simulink model "motorFFT"  (R2024b)
settings: Solver=FixedStepAuto  StartTime=0.0  StopTime=64  FixedStep=15e-3  RelTol=1e-3
libraries: SignalEditorBlockLib x9, spspowerguiLib x1
settings Model: SimulationMode=rapid-accelerator  Creator=Nitesh  LastModifiedBy=Nitesh
settings DataIOCC: ReturnWorkspaceOutputs=off
settings GRTTargetCC: RTWCAPISignals=on  RTWCAPIParams=on

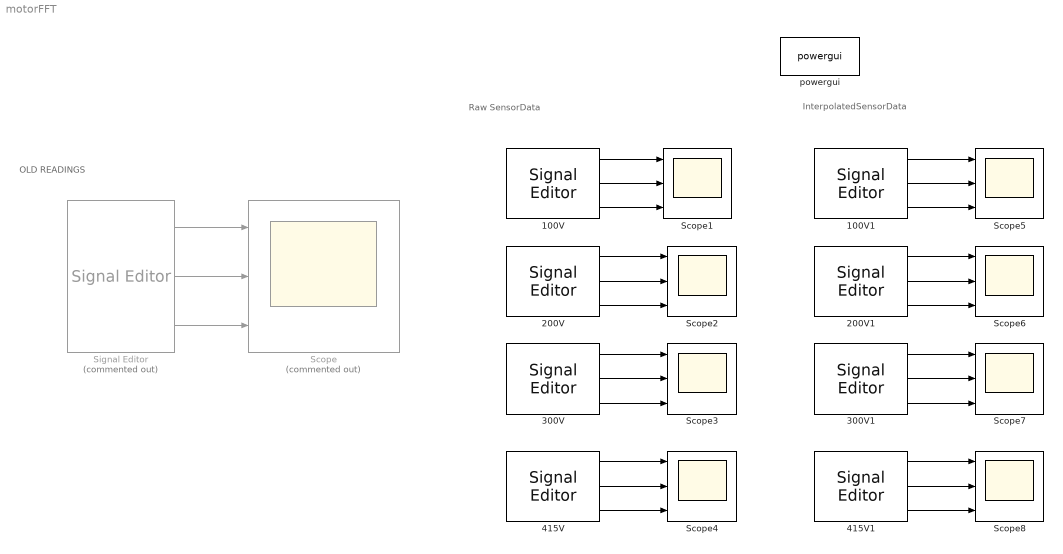
== system motorFFT ==
  note: InterpolatedSensorData
  note: Raw SensorData
  note: OLD READINGS
  100V : SignalEditorBlockLib/Signal Editor  FileName=_100V_scenario.mat  ActiveScenario=scenario  ActiveSignal=Xa  IsBus=off  OutputBusObjectStr=Bus: BusObject  SampleTime=0  Interpolate=off  ZeroCross=off  OutputAfterFinalValue=Setting to zero  Unit=inherit  PreserveSignalName=on  ApplySigPropsToAllScenarios=on  ApplySigPropsToAllSignals=on
  100V1 : SignalEditorBlockLib/Signal Editor  FileName=_100V_scenario.mat  ActiveScenario=scenario  ActiveSignal=Xa  IsBus=off  OutputBusObjectStr=Bus: BusObject  SampleTime=0  ZeroCross=off  OutputAfterFinalValue=Setting to zero  Unit=inherit  PreserveSignalName=on  ApplySigPropsToAllScenarios=on  ApplySigPropsToAllSignals=on
  200V : SignalEditorBlockLib/Signal Editor  FileName=_200V_scenario.mat  ActiveScenario=scenario  ActiveSignal=Xa  IsBus=off  OutputBusObjectStr=Bus: BusObject  SampleTime=0  Interpolate=off  ZeroCross=off  OutputAfterFinalValue=Setting to zero  Unit=inherit  PreserveSignalName=on  ApplySigPropsToAllScenarios=on  ApplySigPropsToAllSignals=on
  200V1 : SignalEditorBlockLib/Signal Editor  FileName=_200V_scenario.mat  ActiveScenario=scenario  ActiveSignal=Xa  IsBus=off  OutputBusObjectStr=Bus: BusObject  SampleTime=0  ZeroCross=off  OutputAfterFinalValue=Setting to zero  Unit=inherit  PreserveSignalName=on  ApplySigPropsToAllScenarios=on  ApplySigPropsToAllSignals=on
  300V : SignalEditorBlockLib/Signal Editor  FileName=_300_scenario.mat  ActiveScenario=scenario  ActiveSignal=Xa  IsBus=off  OutputBusObjectStr=Bus: BusObject  SampleTime=0  Interpolate=off  ZeroCross=off  OutputAfterFinalValue=Setting to zero  Unit=inherit  PreserveSignalName=on  ApplySigPropsToAllScenarios=on  ApplySigPropsToAllSignals=on
  300V1 : SignalEditorBlockLib/Signal Editor  FileName=_300_scenario.mat  ActiveScenario=scenario  ActiveSignal=Xa  IsBus=off  OutputBusObjectStr=Bus: BusObject  SampleTime=0  ZeroCross=off  OutputAfterFinalValue=Setting to zero  Unit=inherit  PreserveSignalName=on  ApplySigPropsToAllScenarios=on  ApplySigPropsToAllSignals=on
  415V : SignalEditorBlockLib/Signal Editor  FileName=_415V_scenario.mat  ActiveScenario=scenario  ActiveSignal=Xa  IsBus=off  OutputBusObjectStr=Bus: BusObject  SampleTime=0  Interpolate=off  ZeroCross=off  OutputAfterFinalValue=Setting to zero  Unit=inherit  PreserveSignalName=on  ApplySigPropsToAllScenarios=on  ApplySigPropsToAllSignals=on
  415V1 : SignalEditorBlockLib/Signal Editor  FileName=_415V_scenario.mat  ActiveScenario=scenario  ActiveSignal=Xa  IsBus=off  OutputBusObjectStr=Bus: BusObject  SampleTime=0  ZeroCross=off  OutputAfterFinalValue=Setting to zero  Unit=inherit  PreserveSignalName=on  ApplySigPropsToAllScenarios=on  ApplySigPropsToAllSignals=on
  Scope : Scope  Commented=on  NumInputPorts=3
  Scope{1..8} (8 alike) : Scope  NumInputPorts=3
  Signal Editor : SignalEditorBlockLib/Signal Editor  Commented=on  FileName=your_scenario_file.mat  ActiveScenario=scenario  ActiveSignal=Xa  IsBus=off  OutputBusObjectStr=Bus: BusObject  SampleTime=0  ZeroCross=off  OutputAfterFinalValue=Setting to zero  Unit=inherit  PreserveSignalName=on  ApplySigPropsToAllScenarios=on  ApplySigPropsToAllSignals=on
  powergui : spspowerguiLib/powergui  Priority=1  SimulationMode=Discrete  SampleTime=50e-6  frequency=60  Iterations=50  frequencyindice=60  Pbase=100e6  ErrMax=1e-4  UnitsV=kV  UnitsW=MW  buscounter=0  FunctionMessages=off  echomessages=off  EnableUseOfTLC=off  CurrentSourceSwitches=off  DisableSnubberDevices=off  DisableRonSwitches=off  DisableVfSwitches=off  DisplayEquations=off  AutomaticDiscreteSolvers=off  SolverType=Tustin/Backward Euler (TBE)  Interpol=off  ExternalGateDelay=off  methode=off  Ts=100  x0status=blocks  SPID=on  SwTol=0  HookPort=off  NonlinearTolerance=1e-4  nMaxIteration=100  ContinueOnMaxIteration=off  RestoreLinks=warning  ResistiveCurrentMeasurement=off  Frange=[0:2:500]  Ylog=off  Xlog=on  ShowGrid=off  save=off  variable=ZData  structure=0  ZoomFFT=off  StartTime=0.0  cycles=1  DisplayStyle=1  fundamental=60  FreqAxis=off  MaxFrequency=1000  frequencyindicesteady=1  RmsSteady=1  display=off
  wires:
  Signal Editor/1 -> Scope/1
  Signal Editor/2 -> Scope/2
  Signal Editor/3 -> Scope/3
  100V/3 -> Scope1/3
  100V/2 -> Scope1/2
  100V/1 -> Scope1/1
  200V/1 -> Scope2/1
  200V/2 -> Scope2/2
  200V/3 -> Scope2/3
  300V/3 -> Scope3/3
  300V/2 -> Scope3/2
  300V/1 -> Scope3/1
  415V/1 -> Scope4/1
  415V/2 -> Scope4/2
  415V/3 -> Scope4/3
  415V1/3 -> Scope8/3
  415V1/2 -> Scope8/2
  415V1/1 -> Scope8/1
  300V1/1 -> Scope7/1
  300V1/2 -> Scope7/2
  300V1/3 -> Scope7/3
  200V1/3 -> Scope6/3
  200V1/2 -> Scope6/2
  200V1/1 -> Scope6/1
  100V1/1 -> Scope5/1
  100V1/2 -> Scope5/2
  100V1/3 -> Scope5/3
